simulink subsystem "Orbit_Analysis"  (R2024b)
settings: Solver=VariableStepAuto  StartTime=0.0  StopTime=10.0  RelTol=1e-3
libraries: simulink_extras x1
settings Model: Creator=cpero  LastModifiedBy=cpero

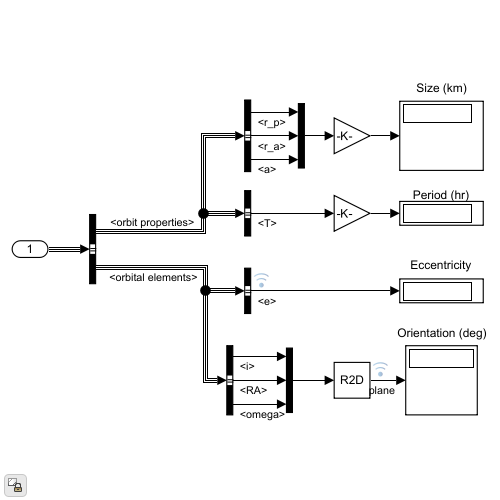
[thumbnail: Simulink's stored preview of the top-level diagram]
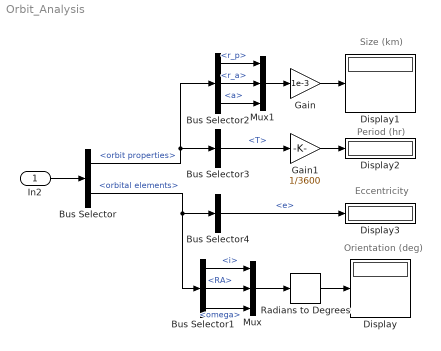
== system Orbit_Analysis ==
  note: Size (km)
  note: Orientation (deg)
  note: Period (hr)
  note: Eccentricity
  In2 : Inport
  Bus Selector : BusSelector  OutputSignals=orbit properties,orbital elements
  Bus Selector1 : BusSelector  OutputSignals=i,RA,omega
  Bus Selector2 : BusSelector  OutputSignals=r_p,r_a,a
  Bus Selector3 : BusSelector  OutputSignals=T
  Bus Selector4 : BusSelector  OutputSignals=e
  Display{,1..3} (4 alike) : Display
  Gain : Gain  Gain=1e-3
  Gain1 : Gain  Gain=1/3600
  Mux : Mux  Inputs=3
  Mux1 : Mux  Inputs=3
  Radians to Degrees : simulink_extras/Transformations/Radians to Degrees
  wires:
  Gain/1 -> Display1/1
  Bus Selector2/3 -> Mux1/3  "<a>"
  Bus Selector1/1 -> Mux/1  "<i>"
  Bus Selector2/2 -> Mux1/2  "<r_a>"
  Mux/1 -> Radians to Degrees/1
  Bus Selector2/1 -> Mux1/1  "<r_p>"
  Bus Selector/2 -> Bus Selector4/1, Bus Selector1/1  "<orbital elements>"
  In2/1 -> Bus Selector/1
  Bus Selector1/3 -> Mux/3  "<omega>"
  Bus Selector4/1 -> Display3/1  "<e>"
  Radians to Degrees/1 -> Display/1
  Bus Selector/1 -> Bus Selector2/1, Bus Selector3/1  "<orbit properties>"
  Bus Selector1/2 -> Mux/2  "<RA>"
  Bus Selector3/1 -> Gain1/1  "<T>"
  Gain1/1 -> Display2/1
  Mux1/1 -> Gain/1
